simulink model "COM_Functional_sl"  (R2016a)
settings: Solver=FixedStepDiscrete  StartTime=0.0  StopTime=10.0  RelTol=1e-3
undefined symbols (not defined in the file): BRAKE_PRESSURE_LO, BRAKE_PRESSURE_MAX, BRAKE_PRESSURE_MED, dt, LO, MANUAL, MAX, MED
libraries: BSCU_lib x3
settings Model: Creator=jliu29  LastModifiedBy=jliu29
settings DataIOCC: LimitDataPoints=on
settings DebuggingCC: AllowSymbolicDim=off
settings ModelReferenceCC: PropagateSignalLabelsOutOfModel=off
settings RTWCC: Description=Generic Real-Time Target
settings GRTTargetCC: GeneratePreprocessorConditionals=Use local settings
settings ConfigComp: DVMode=PropertyProving  DVTestSuiteOptimization=CombinedObjectives (Nonlinear Extended)  DVAssertions=EnableAll  DVProofAssumptions=EnableAll  DVDisplayReport=off

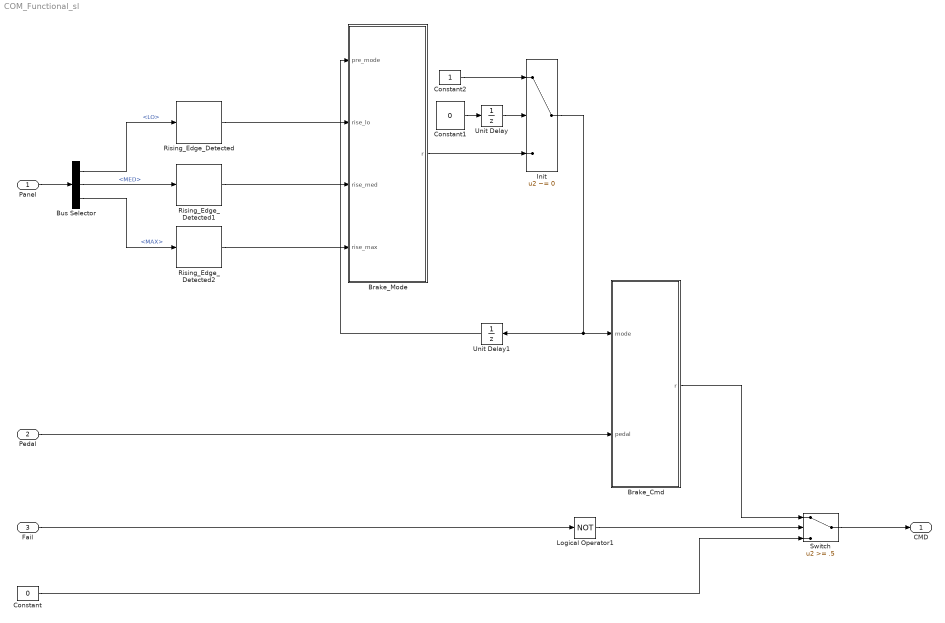
== system COM_Functional_sl ==
  Panel : Inport  OutDataTypeStr=Bus: PanelMsgImpl
  Pedal : Inport  Port=2  OutDataTypeStr=int32  SampleTime=dt  Interpolate=off
  Fail : Inport  Port=3  OutDataTypeStr=boolean  SampleTime=dt  Interpolate=off
  Brake_Cmd : Stateflow chart  TreatAsAtomicUnit=on
  Brake_Mode : Stateflow chart  TreatAsAtomicUnit=on
  Bus Selector : BusSelector  OutputSignals=LO,MED,MAX
  Constant : Constant  Value=0  OutDataTypeStr=int32
  Constant1 : Constant  DisableCoverage=on  Value=0  OutDataTypeStr=boolean
  Constant2 : Constant  OutDataTypeStr=int32
  Init : Switch  Criteria=u2 ~= 0  OutDataTypeStr=Inherit: Inherit via back propagation  ZeroCross=off  InputSameDT=on
  Logical Operator1 : Logic  Operator=NOT  OutDataTypeStr=boolean
  Rising_Edge_Detected : BSCU_lib/Rising_Edge_Detected
  Rising_Edge_Detected1 : BSCU_lib/Rising_Edge_Detected
  Rising_Edge_Detected2 : BSCU_lib/Rising_Edge_Detected
  Switch : Switch  Description=May be used within well defined functions, or functions that soley define logical expressions.  Threshold=.5  ZeroCross=off  InputSameDT=on
  Unit Delay : UnitDelay  InitialCondition=1  SampleTime=-1
      settings: AttributesFormatString=<Init = %<InitialCondition>>
  Unit Delay1 : UnitDelay  InitialCondition=1  SampleTime=-1
      settings: AttributesFormatString=<Init = %<InitialCondition>>
  CMD : Outport  OutDataTypeStr=int32
  wires:
  Panel/1 -> Bus Selector/1
  Brake_Mode/1(r) -> Init/3
  Init/1 -> Unit Delay1/1, Brake_Cmd/1(mode)
  Bus Selector/1 -> Rising_Edge_Detected/1  "<LO>"
  Bus Selector/2 -> Rising_Edge_Detected1/1  "<MED>"
  Bus Selector/3 -> Rising_Edge_Detected2/1  "<MAX>"
  Rising_Edge_Detected/1 -> Brake_Mode/2(rise_lo)
  Rising_Edge_Detected1/1 -> Brake_Mode/3(rise_med)
  Rising_Edge_Detected2/1 -> Brake_Mode/4(rise_max)
  Unit Delay/1 -> Init/2
  Constant1/1 -> Unit Delay/1
  Constant2/1 -> Init/1
  Pedal/1 -> Brake_Cmd/2(pedal)
  Fail/1 -> Logical Operator1/1
  Logical Operator1/1 -> Switch/2
  Constant/1 -> Switch/3
  Brake_Cmd/1(r) -> Switch/1
  Switch/1 -> CMD/1
  Unit Delay1/1 -> Brake_Mode/1(pre_mode)

== stateflow chart COM_Functional_sl/Brake_Cmd ==
  (default) -> (junction 4789)
  (junction 4789) -> (junction 4790) [order 1] : [mode == LO]
  (junction 4789) -> (junction 4791) [order 2]
  (junction 4790) -> (junction 4798) : {
      | r = BRAKE_PRESSURE_LO;
      | }
  (junction 4791) -> (junction 4792) [order 1] : [mode == MED ]
  (junction 4791) -> (junction 4793) [order 2]
  (junction 4792) -> (junction 4797) : {
      | r = BRAKE_PRESSURE_MED;
      | }
  (junction 4793) -> (junction 4794) [order 1] : [mode == MAX]
  (junction 4793) -> (junction 4800) [order 2]
  (junction 4794) -> (junction 4796) : {
      | r = BRAKE_PRESSURE_MAX;
      | }
  (junction 4800) -> (junction 4795) : {
      | r = pedal;
      | }
  (junction 4796) -> (junction 4795)
  (junction 4797) -> (junction 4796)
  (junction 4798) -> (junction 4797)
  (junction 4795) -> (junction 4799)
  data: mode input int32; pedal input int32; r output int32; MANUAL parameter =1; LO parameter =2; MED parameter =3; MAX parameter =4; BRAKE_PRESSURE_LO parameter; BRAKE_PRESSURE_MAX parameter; BRAKE_PRESSURE_MED parameter

== stateflow chart COM_Functional_sl/Brake_Mode ==
  (default) -> (junction 4789)
  (junction 4789) -> (junction 4790) [order 1] : [  ((pre_mode == LO) && rise_lo) || ...
      |    ((pre_mode == MED) && rise_med) || ...
      |    ((pre_mode == MAX) && rise_max)
      | ]
  (junction 4789) -> (junction 4791) [order 2]
  (junction 4790) -> (junction 4798) : {
      | r = MANUAL;
      | }
  (junction 4791) -> (junction 4792) [order 1] : [  (pre_mode != LO) && rise_lo ]
  (junction 4791) -> (junction 4793) [order 2]
  (junction 4792) -> (junction 4797) : {
      | r = LO;
      | }
  (junction 4793) -> (junction 4794) [order 1] : [ (pre_mode != MED) && rise_med ]
  (junction 4793) -> (junction 4800) [order 2]
  (junction 4794) -> (junction 4796) : {
      | r = MED;
      | }
  (junction 4800) -> (junction 4808) [order 1] : [ (pre_mode != MAX) && rise_max ]
  (junction 4800) -> (junction 4795) [order 2] : {
      | r = pre_mode;
      | }
  (junction 4808) -> (junction 4810) : {
      | r = MAX;
      | }
  (junction 4810) -> (junction 4795)
  (junction 4796) -> (junction 4810)
  (junction 4797) -> (junction 4796)
  (junction 4798) -> (junction 4797)
  (junction 4795) -> (junction 4799)
  data: pre_mode input int32; rise_lo input boolean; rise_med input boolean; rise_max input boolean; r output int32; MANUAL parameter =1; LO parameter =2; MED parameter =3; MAX parameter =4
